simulink model "FIR_MAC32"  (Simulink 6.3)
settings: Solver=VariableStepDiscrete  StartTime=0.0  StopTime=5000 * FilterRate  FixedStep=FilterRate  RelTol=1e-3
PreLoadFcn:
  | close all
  | coef = fix(fir1(32,3/8)*2^16-1);
  | Impulse =  zeros(1,1000);
  | Impulse(1) = 1;
  | h = conv(coef,Impulse);
  | plot(coef,'o');
  | title('Fixed-point scaled coefficient value');
  | fftplot(h);
  | title('Impulse Frequency response');
  | SymbolRate = 1 / 1e6;
  | FilterRate = SymbolRate / 32;
InitFcn:
  | SymbolRate = 1 / 1e6
  | FilterRate = SymbolRate / 32
  | %% DSPBuilder Start
  | alt_dspbuilder_update_model(bdroot)
  | %% DSPBuilder End
StartFcn:
  | SymbolRate = 1 / 1e6;
  | FilterRate = SymbolRate / 32;
libraries: allblocks_alteradspbuilder2 x20, simulink x1
settings Model: Creator=mjervis  LastModifiedBy=LKONG
settings DataIOCC: SignalLoggingName=sigsOut
settings OptimizationCC: InlineInvariantSignals=on
settings DebuggingCC: SolverPrmCheckMsg=none
settings HardwareCC: TargetUnknown=on

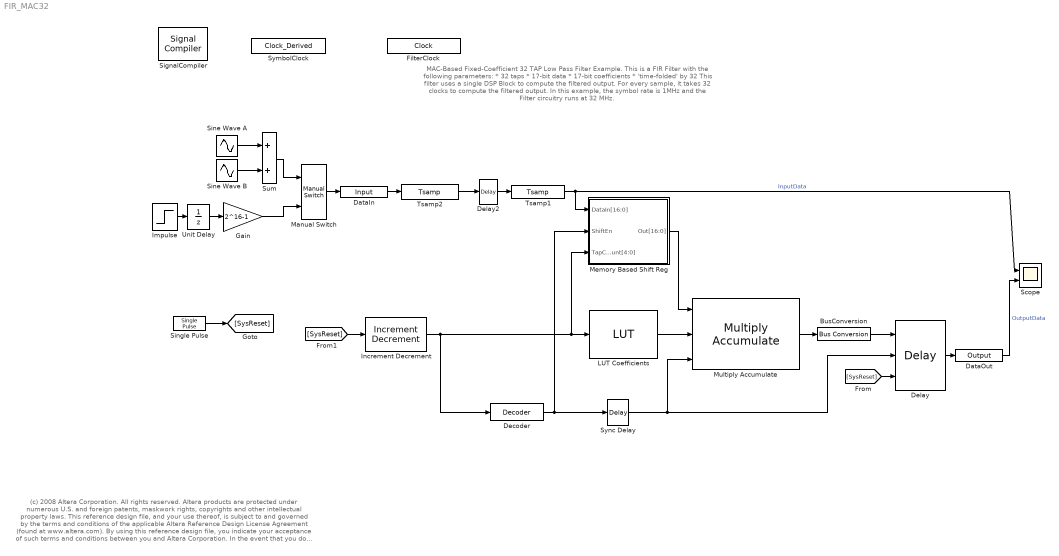
== system FIR_MAC32 ==
  note: MAC-Based Fixed-Coefficient 32 TAP Low Pass Filter Example.
      | This is a FIR Filter with the following parameters:
      |   * 32 taps
      |   * 17-bit data
      |   * 17-bit coefficients
      |   * 'time-folded' by 32
      | This filter uses a single DSP Block to compute the filtered output. For every sample,
      | it takes 32 clocks to compute the filtered output. In this example, the symbol rate
      | is 1MHz and the Filter circuitry runs at 32 MHz.
  note: (c) 2008 Altera Corporation. All rights reserved.  Altera products are protected under numerous U.S. and foreign patents, maskwork rights, copyrights and other intellectual property laws.
      | This reference design file, and your use thereof, is subject to and governed by the terms and conditions of the applicable Altera Reference Design License Agreement (found at www.altera.com).
      | By using this reference design file, you indicate your acceptance of such terms and conditions between you and Altera Corporation.
      | In the event that you do not agree with such terms and conditions, you may not use the reference design file and please promptly destroy any copies you have made.
      | This reference design file being provided on an "as-is" basis and as an accommodation and therefore all warranties, representations or guarantees of any kind (whether express, implied or statutory)
      | including, without limitation, warranties of merchantability, non-infringement, or fitness for a particular purpose, are specifically disclaimed.
      | By making this reference design file available, Altera expressly does not recommend, suggest or require that this reference design file be used in combination with any other product not provided by Altera
  BusConversion : allblocks_alteradspbuilder2/Bus Conversion  BusType=Signed Integer  ibwl=34  ibwr=0  bwl=17  bwr=0  bitToConnectToOutputLSB=17  round=off  saturate=off
  DataIn : allblocks_alteradspbuilder2/Input  iofile=d:\wsTrunk\workspace\Documentation\DesignExamples\Demos\Filters\Mac32\tb_FIR_MAC32\FIR_MAC32_DataIn.salt  BusType=Signed Integer  bwl=17  bwr=0  SpecifyClock=on  clock=SymbolClock  PORTTYPE=Input
  DataOut : allblocks_alteradspbuilder2/Output  iofile=d:\wsTrunk\workspace\Documentation\DesignExamples\Demos\Filters\Mac32\tb_FIR_MAC32\FIR_MAC32_DataOut.capture  BusType=Signed Integer  bwl=18  bwr=0  PORTTYPE=Output
  Decoder : allblocks_alteradspbuilder2/Decoder  BusType=Unsigned Integer  bwl=5  bwr=0  registered=off  value=1
  Delay : allblocks_alteradspbuilder2/Delay  pipeline=1  ClockPhase=1  use_ena=on  use_sclr=on  use_init=off  reset_value=1
  Delay2 : allblocks_alteradspbuilder2/Delay  pipeline=1  ClockPhase=1  use_ena=off  use_sclr=off  use_init=off  reset_value=1
  FilterClock : allblocks_alteradspbuilder2/Clock  ClockPeriod=31.25  ClockPeriodUnit=ns  SampleTime=3.125e-008  SimulationStartCycle=5  PhaseOffset=0  Reset=aclr  ResetType=Active Low  Export=off
  Gain : Gain  Gain=2^16-1  SaturateOnIntegerOverflow=on
  Impulse : Step  Time=SymbolRate  Before=1  After=0  SampleTime=SymbolRate
  Increment Decrement : allblocks_alteradspbuilder2/Increment Decrement  BusType=Unsigned Integer  bwl=5  bwr=0  SpecifyClock=off  clr_value=0  direction=Increment  phase_selection=1  use_ena=off  use_sclr=on
  LUT Coefficients : allblocks_alteradspbuilder2/LUT  addr_width=5  BusType=Signed Integer  bwl=17  bwr=0  init_array=(fir1(31,3/8)) .* 2^16-1  use_ena=off  reg_data=off  use_lpm=on  reg_addr=on  ram_type=AUTO
  Manual Switch : simulink/Signal Routing/Manual Switch  sw=0  action=0
  Memory Based Shift Reg : Subsystem  AncestorBlock=shift_reg/Memory Based Shift Reg
      mask Type: SubSystem AlteraBlockSet
  Multiply Accumulate : allblocks_alteradspbuilder2/Multiply Accumulate  BusType=Signed Integer  abwl=17  abwr=0  bbwl=17  bbwr=0  ywidth=34  pipeline_register=Data Inputs and Multiplier  direction=Add  use_addsub=off  use_ena=off  use_aclr=off  UseDedicatedCircuitry=AUTO
  Scope : Scope  NumInputPorts=2
      settings: TimeRange=0.00016  YMin=-25000~-15000  YMax=25000~15000
  SignalCompiler : allblocks_alteradspbuilder2/Signal Compiler  DeviceFamily=Stratix III  DeviceName=AUTO  EnableSignalTap=off  SignalTapDepth=128  UseBoardBlock=off  StpUseDefaultClock=on  StpClock=clock
  Sine Wave A : Sin  SineType=Sample based  Amplitude=2^14-1  Frequency=2*pi*100e3  Samples=floor (2*pi / (250e3 * SymbolRate))  SampleTime=SymbolRate
  Sine Wave B : Sin  SineType=Sample based  Amplitude=2^13-1  Frequency=2*pi*100e3  Samples=floor (2*pi / (100e3* SymbolRate))  SampleTime=SymbolRate
  "Single Pulse " : allblocks_alteradspbuilder2/Single Pulse  signal_type=Step Down  impulse_width=1  delay=2  SpecifyClock=off  use_ena=off  use_sclr=off
  Sum : Sum  SaturateOnIntegerOverflow=on  InputSameDT=on
  SymbolClock : allblocks_alteradspbuilder2/Clock_Derived  ClockNumerator=32  ClockDenominator=1  SimulationStartCycle=5  PhaseOffset=0  Reset=aclr1  ResetType=Active Low  Export=off
  Sync Delay : allblocks_alteradspbuilder2/Delay  pipeline=2  ClockPhase=1  use_ena=off  use_sclr=off  use_init=off  reset_value=1
  Tsamp1 : allblocks_alteradspbuilder2/Tsamp  SpecifyClock=off  clock=Clock
  Tsamp2 : allblocks_alteradspbuilder2/Tsamp  SpecifyClock=on  clock=SymbolClock
  Unit Delay : UnitDelay  SampleTime=-1
  wires:
  Increment Decrement/1 -> Decoder/1, Memory Based Shift Reg/3(TapCount[4:0]), LUT Coefficients/1
  DataIn/1 -> Tsamp2/1
  Multiply Accumulate/1 -> BusConversion/1
  Sine Wave A/1 -> Sum/1
  Sine Wave B/1 -> Sum/2
  Delay/1 -> DataOut/1
  [SysReset] -> Delay/3
  BusConversion/1 -> Delay/1
  Memory Based Shift Reg/1(Out[16:0]) -> Multiply Accumulate/1
  Delay2/1 -> Tsamp1/1
  Tsamp1/1 -> Memory Based Shift Reg/1(DataIn[16:0]), Scope/1  "InputData"
  Sync Delay/1 -> Delay/2, Multiply Accumulate/3
  LUT Coefficients/1 -> Multiply Accumulate/2
  [SysReset] -> Increment Decrement/1
  Gain/1 -> Manual Switch/2
  Manual Switch/1 -> DataIn/1
  Sum/1 -> Manual Switch/1
  DataOut/1 -> Scope/2  "OutputData"
  Decoder/1 -> Sync Delay/1, Memory Based Shift Reg/2(ShiftEn)
  Tsamp2/1 -> Delay2/1
  Impulse/1 -> Unit Delay/1
  Unit Delay/1 -> Gain/1
  "Single Pulse "/1 -> [SysReset]

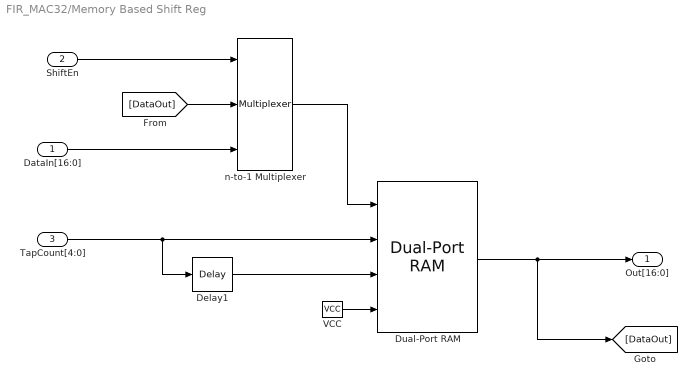
== system FIR_MAC32/Memory Based Shift Reg ==
  DataIn[16:0] : Inport
  ShiftEn : Inport  Port=2
  TapCount[4:0] : Inport  Port=3
  Delay1 : allblocks_alteradspbuilder2/Delay  pipeline=1  ClockPhase=1  use_ena=off  use_sclr=off  use_init=off  reset_value=1
  Dual-Port RAM : allblocks_alteradspbuilder2/Dual-Port RAM  numwords=2^(5)  BusType=Inferred  bwl=8  bwr=0  memory_type=AUTO  ram_type=DualRAM  initialization=Blank  init_file=input.hex  init_array=[0:1:15]  register_outputs=on  use_ena=off  ClockPhase=1
  VCC : allblocks_alteradspbuilder2/VCC  SpecifyClock=off
  n-to-1 Multiplexer : allblocks_alteradspbuilder2/Multiplexer  numInputs=2  pipeline=0  oneHot=off  use_ena=off  use_aclr=off
  Out[16:0] : Outport
  wires:
  [DataOut] -> n-to-1 Multiplexer/2
  n-to-1 Multiplexer/1 -> Dual-Port RAM/1
  Dual-Port RAM/1 -> [DataOut], Out[16:0]/1
  VCC/1 -> Dual-Port RAM/4
  DataIn[16:0]/1 -> n-to-1 Multiplexer/3
  ShiftEn/1 -> n-to-1 Multiplexer/1
  TapCount[4:0]/1 -> Delay1/1, Dual-Port RAM/2
  Delay1/1 -> Dual-Port RAM/3
